simulink model "pm_motor"  (R2018a)
settings: Solver=VariableStepAuto  StartTime=0.0  StopTime=10.0  RelTol=1e-3
values from neighbouring files (symbols this model uses):
  Bm = 6.04e-6    (= 6.04e-06)    [pm_par.m]    (also in series_par.m)
  J = 1    [dc_par.m]    (also in pm_par.m = 2.12e-06; series_par.m = 2.12e-06)
  Kv = 1.41e-2    (= 0.0141)    [pm_par.m]
  Ra = 0.6    [dc_par.m]    (also in pm_par.m = 7; series_par.m = 6)
  Ta = La/Ra    (= 0.02)    [dc_par.m]    (also in pm_par.m = 0.0171428571429)
  Tm = 29    [dc_par.m]    (also in pm_par.m = 0.00353; series_par.m = 0.00353)
  Va = 240    [dc_par.m]    (also in pm_par.m = 6; series_par.m = 6)
settings Model: Creator=Jasper  LastModifiedBy=jasper

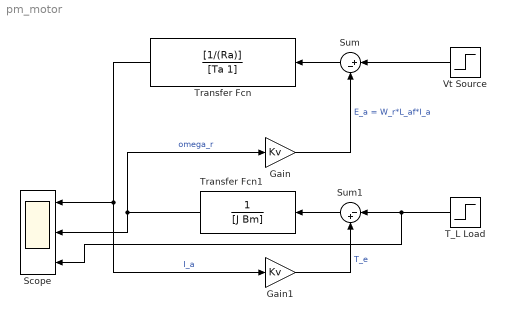
== system pm_motor ==
  Gain : Gain  Gain=Kv
  Gain1 : Gain  Gain=Kv
  Scope : Scope  NumInputPorts=3
  Sum : Sum  Inputs=|+-
  Sum1 : Sum  Inputs=|-+
  T_L Load : Step  Time=4  After=Tm*0.25  SampleTime=0
  Transfer Fcn : TransferFcn  Numerator=[1/(Ra)]  Denominator=[Ta 1]
  Transfer Fcn1 : TransferFcn  Denominator=[J Bm]
  Vt Source : Step  Time=0  Before=Va*3  After=Va*3  SampleTime=0
  wires:
  Gain/1 -> Sum/2  "E_a = W_r*L_af*I_a"
  Vt Source/1 -> Sum/1
  Sum/1 -> Transfer Fcn/1
  Transfer Fcn/1 -> Gain1/1, Scope/1  "I_a"
  Transfer Fcn1/1 -> Gain/1, Scope/2  "omega_r"
  Sum1/1 -> Transfer Fcn1/1
  Gain1/1 -> Sum1/2  "T_e"
  T_L Load/1 -> Scope/3, Sum1/1
